simulink model "gmaw_process"  (R2021a)
settings: Solver=ode1  StartTime=0.0  StopTime=0.001  FixedStep=1e-09  RelTol=1e-3
values from neighbouring files (symbols this model uses):
  alpha = 7.79*10^(-6)    (= 7.79e-06)    [init_params.m]
  Aw = pi*rw^2    (= 1.13097335529e-06)    [init_params.m]
  C1 = 3.2634*10^(-10)    (= 3.2634e-10)    [init_params.m]
  C2 = 1.1836*10^(-9)    (= 1.1836e-09)    [init_params.m]
  DeltaT = 1300    [init_params.m]
  Ea = 723.2561    [init_params.m]
  k = 24    [init_params.m]
  kv = 10    [init_params.m]
  lc = 0.01    [init_params.m]
  Ls = 0.00014    [init_params.m]
  n = 0.655    [init_params.m]
  nd = 0.958    [init_params.m]
  Ra = 0.0201    [init_params.m]
  rho = 0.1319    [init_params.m]
  Rs = 0.004    [init_params.m]
  v = 0.12    [init_params.m]
  Vo = 5.1782    [init_params.m]
  Voc = 31    [init_params.m]
undefined symbols (not defined in the file or in its folder): sigbuilder_block
settings Model: PacingRate=0.010000  Creator=igor  LastModifiedBy=lucas

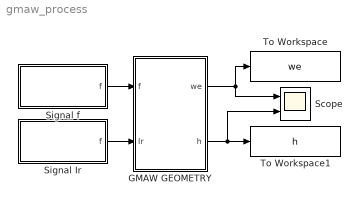
== system gmaw_process ==
  GMAW GEOMETRY : Subsystem
  Scope : Scope  NumInputPorts=2
  Signal Ir : Subsystem  Tag=STV Subsys  LoadFcn=sigbuilder_block('load');  StartFcn=sigbuilder_block('start');  StopFcn=sigbuilder_block('stop');  ClipboardFcn=sigbuilder_block('clipboard');  mask(Sigbuilder block){tuvar=[0:10]}
      mask help: Simulink:masks:SigbuilderBlock_MD
      mask init:
      | if ~strcmp(get_param(bdroot(gcbh),'SimulationStatus'),'stopped') tuvar = sigbuilder_block('maskInit'); end
      settings: CopyFcn=sigbuilder_block('copy');  DeleteFcn=sigbuilder_block('delete');  ModelCloseFcn=sigbuilder_block('modelClose');  PreSaveFcn=sigbuilder_block('preSave');  PauseFcn=sigbuilder_block('pause');  ContinueFcn=sigbuilder_block('continue');  NameChangeFcn=sigbuilder_block('namechange');  OpenFcn=sigbuilder_block('open',[533.25 126 1213.5 399.75 ]);  CloseFcn=sigbuilder_block('close');
      mask Display: plot(0, 0, 100, 100,[2, 2, 32, 32, 2], [68, 8, 8, 68, 68],[32, 2], [38, 38], [32, 19, 2],[53, 60, 44], [32, 17, 17, 2],[16, 16, 31, 31]);txt = getActiveGroup(gcbh);text(2, 100, txt,'verticalAlignment', 'top');
  Signal f : Subsystem  Tag=STV Subsys  LoadFcn=sigbuilder_block('load');  StartFcn=sigbuilder_block('start');  StopFcn=sigbuilder_block('stop');  ClipboardFcn=sigbuilder_block('clipboard');  mask(Sigbuilder block){tuvar=[0:10]}
      mask help: Simulink:masks:SigbuilderBlock_MD
      mask init:
      | if ~strcmp(get_param(bdroot(gcbh),'SimulationStatus'),'stopped') tuvar = sigbuilder_block('maskInit'); end
      settings: CopyFcn=sigbuilder_block('copy');  DeleteFcn=sigbuilder_block('delete');  ModelCloseFcn=sigbuilder_block('modelClose');  PreSaveFcn=sigbuilder_block('preSave');  PauseFcn=sigbuilder_block('pause');  ContinueFcn=sigbuilder_block('continue');  NameChangeFcn=sigbuilder_block('namechange');  OpenFcn=sigbuilder_block('open',[6 30 1908 681.75 ]);  CloseFcn=sigbuilder_block('close');
      mask Display: plot(0, 0, 100, 100,[2, 2, 32, 32, 2], [68, 8, 8, 68, 68],[32, 2], [38, 38], [32, 19, 2],[53, 60, 44], [32, 17, 17, 2],[16, 16, 31, 31]);txt = getActiveGroup(gcbh);text(2, 100, txt,'verticalAlignment', 'top');
  To Workspace : ToWorkspace  VariableName=we  SaveFormat=Timeseries  SampleTime=-1
  To Workspace1 : ToWorkspace  VariableName=h  SaveFormat=Timeseries  SampleTime=-1
  wires:
  Signal Ir/1(f) -> GMAW GEOMETRY/2(Ir)
  GMAW GEOMETRY/1(we) -> To Workspace/1, Scope/1
  GMAW GEOMETRY/2(h) -> Scope/2, To Workspace1/1
  Signal f/1(f) -> GMAW GEOMETRY/1(f)

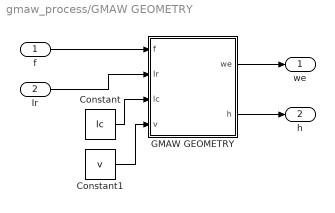
== system gmaw_process/GMAW GEOMETRY ==
  f : Inport
  Ir : Inport  Port=2
  Constant : Constant  Value=lc
  Constant1 : Constant  Value=v
  GMAW GEOMETRY : Subsystem
  we : Outport
  h : Outport  Port=2
  wires:
  Constant/1 -> GMAW GEOMETRY/3(lc)
  GMAW GEOMETRY/2(h) -> h/1
  Constant1/1 -> GMAW GEOMETRY/4(v)
  f/1 -> GMAW GEOMETRY/1(f)
  GMAW GEOMETRY/1(we) -> we/1
  Ir/1 -> GMAW GEOMETRY/2(Ir)

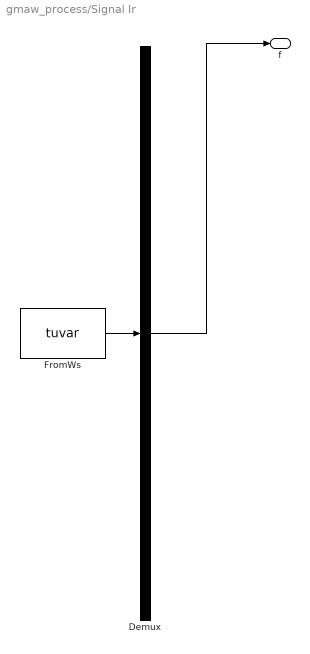
== system gmaw_process/Signal Ir ==
  Demux : Demux  Tag=STV Demux  Outputs=1
      settings: DisplayOption=none
  FromWs : FromWorkspace  Tag=STV FromWs  VariableName=tuvar
      SigBuilderData=|
      | common.afterFinalStr = 'Extrapolate'
      | common.sampleTime = 0
      | dataSet.timeRange = [0 0.001]
      | dataSet.name = 'Ir'
      | sbobj.Groups.Name = 'Ir'
      | sbobj.Groups.Signals.Name = 'f'
      | sbobj.Groups.Signals.XData = [0 1e-06 2e-06 3e-06 4e-06 5e-06 6e-06 7e-06 8e-06 9e-06 1e-05 1.1e-05 ... (1001 elements, 1x1001)]
      | sbobj.Groups.Signals.YData = [113.555555556 133.022222222 94.0888888889 87.6 133.022222222 113.555555556 146 146 100.577777778 94.0888888889 100.577777778 126.533333333 ... (1001 elements, 1x1001)]
      | sbobj.Groups.TimeRange = [0 0.001]
  f : Outport  Tag=STV Outport
  wires:
  FromWs/1 -> Demux/1
  Demux/1 -> f/1

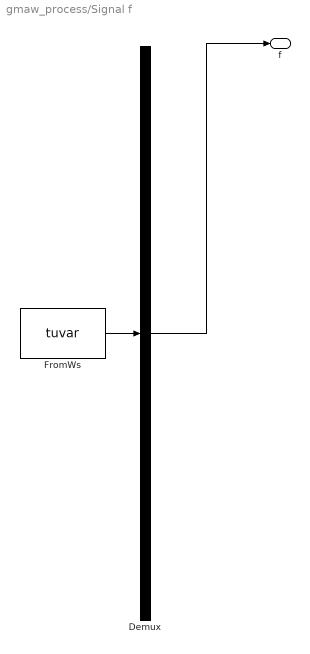
== system gmaw_process/Signal f ==
  Demux : Demux  Tag=STV Demux  Outputs=1
      settings: DisplayOption=none
  FromWs : FromWorkspace  Tag=STV FromWs  VariableName=tuvar
      SigBuilderData=|
      | common.afterFinalStr = 'Extrapolate'
      | common.sampleTime = 0
      | dataSet.timeRange = [0 0.001]
      | dataSet.name = 'f'
      | sbobj.Groups.Name = 'f'
      | sbobj.Groups.Signals.Name = 'f'
      | sbobj.Groups.Signals.XData = [0 1e-06 2e-06 3e-06 4e-06 5e-06 6e-06 7e-06 8e-06 9e-06 1e-05 1.1e-05 ... (1001 elements, 1x1001)]
      | sbobj.Groups.Signals.YData = [0.00611111111111 0.0427777777778 0.0244444444444 0.00611111111111 0.0488888888889 0 0.0305555555556 0.00611111111111 0.0122222222222 0.0183333333333 0.0183333333333 0.0244444444444 ... (1001 elements, 1x1001)]
      | sbobj.Groups.TimeRange = [0 0.001]
  f : Outport  Tag=STV Outport
  wires:
  FromWs/1 -> Demux/1
  Demux/1 -> f/1

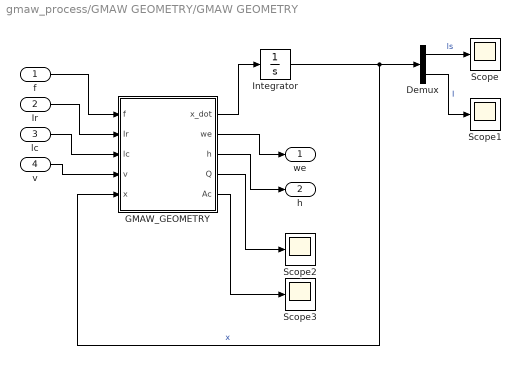
== system gmaw_process/GMAW GEOMETRY/GMAW GEOMETRY ==
  f : Inport
  Ir : Inport  Port=2
  lc : Inport  Port=3
  v : Inport  Port=4
  Demux : Demux  Outputs=2
  GMAW_GEOMETRY : MATLAB Function  TreatAsAtomicUnit=on
  Integrator : Integrator  InitialCondition=[0;0]
  Scope{,1..3} (4 alike) : Scope
  we : Outport
  h : Outport  Port=2
  wires:
  lc/1 -> GMAW_GEOMETRY/3(lc)
  GMAW_GEOMETRY/3(h) -> h/1
  GMAW_GEOMETRY/1(x_dot) -> Integrator/1
  v/1 -> GMAW_GEOMETRY/4(v)
  Ir/1 -> GMAW_GEOMETRY/2(Ir)
  GMAW_GEOMETRY/2(we) -> we/1
  f/1 -> GMAW_GEOMETRY/1(f)
  Integrator/1 -> Demux/1, GMAW_GEOMETRY/5(x)  "x"
  Demux/1 -> Scope/1  "ls"
  Demux/2 -> Scope1/1  "I"
  GMAW_GEOMETRY/4(Q) -> Scope2/1
  GMAW_GEOMETRY/5(Ac) -> Scope3/1

== matlab function gmaw_process/GMAW GEOMETRY/GMAW GEOMETRY/GMAW_GEOMETRY ==
  data: f input; x_dot output; Ir input; lc input; v input; we output; h output; x input; C1 parameter; C2 parameter; DeltaT parameter; rho parameter; Aw parameter; kv parameter; Ra parameter; Rs parameter; Voc parameter; Vo parameter; Ea parameter; Ls parameter; n parameter; nd parameter; k parameter; alpha parameter; Q output; Ac output
function [x_dot, we, h, Q, Ac] = GMAW(f, Ir, lc, v, x, C1, C2, DeltaT, rho, Aw, kv, Ra, Rs, Voc, Vo, Ea, Ls, n, nd, k, alpha)
%% GMAW PROCESS
ls = x(1);
I = x(2);

x1_dot = f - (C2*rho*ls*I^2 + C1*I)/Aw;
x2_dot = (kv*Ir - (Ra + Rs + rho*ls + kv)*I + (Voc - Vo) - Ea*(lc-ls))/Ls;

x_dot = [x1_dot; x2_dot];

Q = n*(Ra*I^2 + (Ea*(lc-ls) + Vo)*I);
Ac = (C2*rho*ls*I^2 + C1*I)/v;

%% GEOMETRY
kw = sqrt((2 - nd)/nd);

we = sqrt((0.4*alpha/(kw*v))^2 - (2*Ac/(kw^2+1) - Q*alpha/(k*DeltaT*v))/kw) - 0.4*alpha/(kw*v);
h = nd*Ac/we;
